simulink model "PHC_Workflow"  (R2026a)
settings: Solver=VariableStepAuto  StopTime=480
undefined symbols (not defined in the file): exprnd

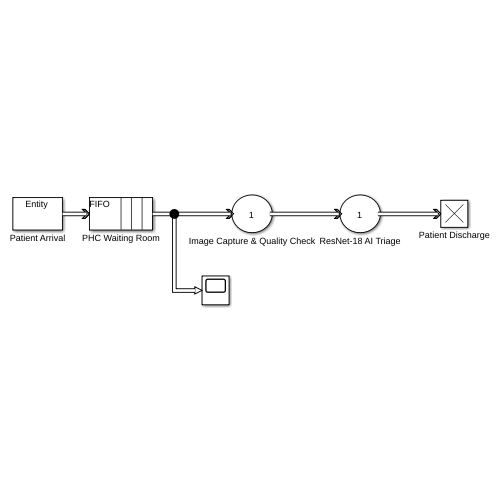
[thumbnail: Simulink's stored preview of the top-level diagram]
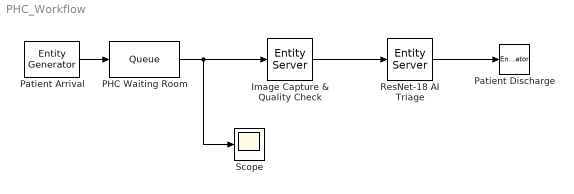
== system PHC_Workflow ==
  Image Capture & Quality Check : EntityServer  InputPortMessageModes=m  OutputPortMessageModes=m  Capacity=1  ServiceTimeValue=3.0
  PHC Waiting Room : Queue  InputPortMessageModes=m  OutputPortMessageModes=m  Capacity=100
  Patient Arrival : EntityGenerator  OutputPortMessageModes=m  Period=exprnd(10)  EntityType=Structured  EntityTypeName=Entity
  Patient Discharge : EntityTerminator  InputPortMessageModes=m
  ResNet-18 AI Triage : EntityServer  InputPortMessageModes=m  OutputPortMessageModes=m  Capacity=1  ServiceTimeValue=0.5
  Scope : Scope
      settings: ActiveDisplayYMinimum=0.9  ActiveDisplayYMaximum=1.1
  wires:
  Patient Arrival/1 -> PHC Waiting Room/1
  Image Capture & Quality Check/1 -> ResNet-18 AI Triage/1
  PHC Waiting Room/1 -> Scope/1, Image Capture & Quality Check/1
  ResNet-18 AI Triage/1 -> Patient Discharge/1
